simulink model "sampleModel2079"  (R2023a)
settings: Solver=VariableStepAuto  StartTime=0.0  StopTime=10.0  RelTol=1e-3
libraries: hdlsllib x8, simulink x3
settings Model: Creator=user1  LastModifiedBy=user1

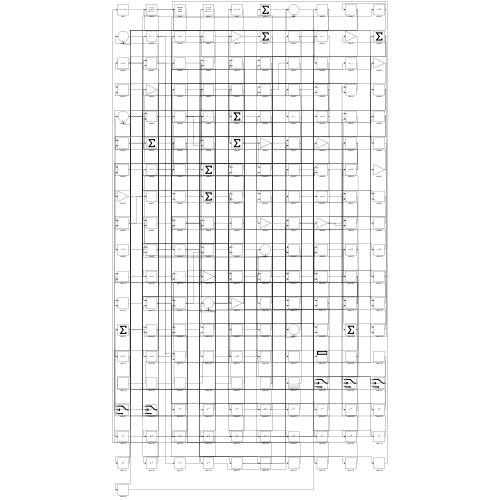
[thumbnail: Simulink's stored preview of the top-level diagram]
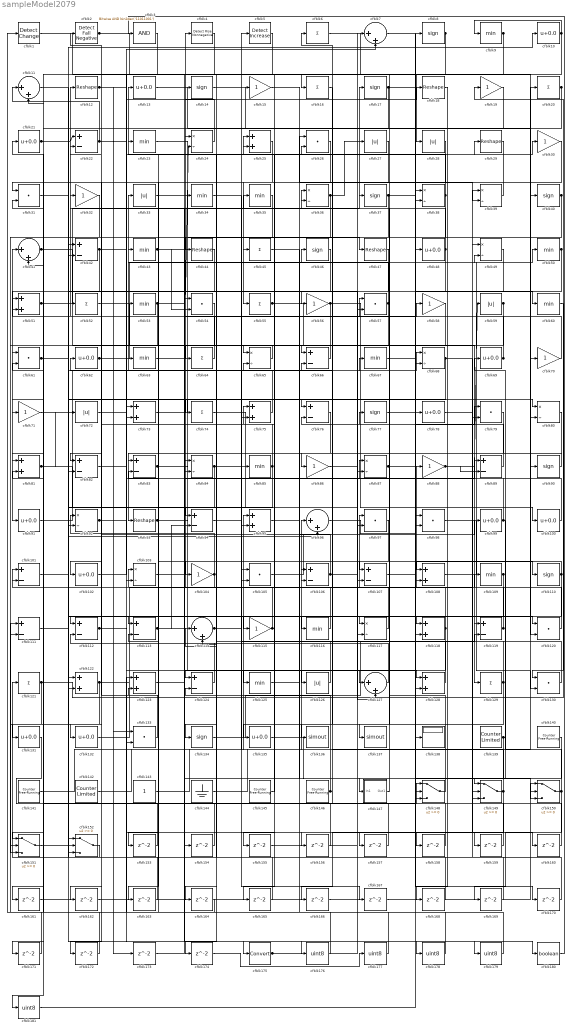
== system sampleModel2079 ==
  cfblk1 : simulink/Logic and Bit Operations/Detect Change  vinit=0  OutDataTypeStr=boolean
      settings: LibrarySourceBlock=|
      | hdlsllib/Logic and Bit
      | Operations/Detect
      | Change
  cfblk{10,13,21,48,62,69,78,91,99..100,102,131..132,135} (14 alike) : Bias  Bias=0.0  SaturateOnIntegerOverflow=off
  cfblk{22,42,66,76,82..83,89,94,101,106..107,111..113,119,124} (16 alike) : Sum  Inputs=+-
  cfblk{24,36,38..39,49,65,68,80,84,87,92,103,117} (13 alike) : Product  Inputs=*/  RndMeth=Zero  SaturateOnIntegerOverflow=on
  cfblk{15,19,30,32,56,58,70..71,86,88,104,115} (12 alike) : Gain
  cfblk{26,31,54,57,61,79,97..98,105,120,130,133} (12 alike) : DotProduct  OutDataTypeStr=Inherit: Inherit via internal rule
  cfblk{25,51,73,75,81,95,108,118,122..123,128} (11 alike) : Sum
  cfblk{9,23,34..35,43,50,53,60,63,67,85,109,116,125} (14 alike) : MinMax
  cfblk{7,11,41,96,114,127} (6 alike) : Sum  Inputs=|++
  cfblk{8,14,17,37,40,46,77,90,110,134} (10 alike) : Signum
  cfblk{12,18,29,44,47,93} (6 alike) : Reshape
  cfblk{6,16,20,45,52,55,64,74,121,129} (10 alike) : Sum  Inputs=+
  cfblk{27..28,33,59,72,126} (6 alike) : Abs  SaturateOnIntegerOverflow=off
  cfblk136 : ToWorkspace  VariableName=simout  SaveFormat=Timeseries  SampleTime=-1
  cfblk137 : ToWorkspace  VariableName=simout  SaveFormat=Timeseries  SampleTime=-1
  cfblk138 : Display
  cfblk139 : hdlsllib/Sources/Counter Limited  uplimit=7  tsamp=-1
  cfblk{140..141,145..146} (4 alike) : hdlsllib/Sources/Counter Free-Running  NumBits=16  tsamp=-1
  cfblk142 : hdlsllib/Sources/Counter Limited  uplimit=7  tsamp=-1
  cfblk143 : Constant  SampleTime=-1
  cfblk144 : Ground
  cfblk147 : Subsystem
      settings: LibrarySourceBlock=|
      | hdlsllib/Ports &
      | Subsystems/Subsystem
  cfblk{148..152} (5 alike) : Switch  SaturateOnIntegerOverflow=off  InputSameDT=off
  cfblk{153..174} (22 alike) : Delay  SampleTime=1
  cfblk175 : DataTypeConversion  SaturateOnIntegerOverflow=off  RndMeth=Floor
  cfblk{176..179,181} (5 alike) : DataTypeConversion  OutDataTypeStr=uint8  SaturateOnIntegerOverflow=off  RndMeth=Floor
  cfblk180 : DataTypeConversion  OutDataTypeStr=boolean  SaturateOnIntegerOverflow=off  RndMeth=Floor
  cfblk2 : hdlsllib/Logic and Bit Operations/Detect Fall Negative  vinit=0  OutDataTypeStr=boolean
  cfblk3 : simulink/Logic and Bit Operations/Bitwise Operator  logicop=AND  UseBitMask=on  BitMask=bin2dec('11011001')  BitMaskRealWorld=Stored Integer
      settings: LibrarySourceBlock=|
      | hdlsllib/Logic and Bit
      | Operations/Bitwise
      | Operator
  cfblk4 : hdlsllib/Logic and Bit Operations/Detect Rise Nonnegative  vinit=0  OutDataTypeStr=boolean
  cfblk5 : simulink/Logic and Bit Operations/Detect Increase  vinit=0.0  OutDataTypeStr=boolean
      settings: LibrarySourceBlock=|
      | hdlsllib/Logic and Bit
      | Operations/Detect
      | Increase
  wires:
  cfblk64/1 -> cfblk12/1
  cfblk76/1 -> cfblk93/1
  cfblk126/1 -> cfblk103/1
  cfblk119/1 -> cfblk97/1, cfblk53/1
  cfblk57/1 -> cfblk33/1, cfblk76/1
  cfblk128/1 -> cfblk62/1
  cfblk70/1 -> cfblk41/1
  cfblk116/1 -> cfblk4/1
  cfblk42/1 -> cfblk91/1, cfblk7/2
  cfblk121/1 -> cfblk19/1, cfblk151/2, cfblk68/2
  cfblk141/1 -> cfblk95/1
  cfblk122/1 -> cfblk88/1, cfblk131/1
  cfblk25/1 -> cfblk112/1
  cfblk48/1 -> cfblk17/1, cfblk135/1
  cfblk23/1 -> cfblk128/1
  cfblk56/1 -> cfblk100/1, cfblk134/1
  cfblk93/1 -> cfblk117/1, cfblk158/1
  cfblk1/1 -> cfblk16/1
  cfblk131/1 -> cfblk148/1
  cfblk40/1 -> cfblk137/1, cfblk151/3
  cfblk89/1 -> cfblk6/1
  cfblk102/1 -> cfblk87/1
  cfblk108/1 -> cfblk50/1
  cfblk88/1 -> cfblk59/1, cfblk89/2
  cfblk65/1 -> cfblk64/1
  cfblk74/1 -> cfblk117/2
  cfblk10/1 -> cfblk9/1, cfblk11/2
  cfblk105/1 -> cfblk98/1
  cfblk38/1 -> cfblk13/1, cfblk44/1, cfblk151/1
  cfblk110/1 -> cfblk115/1, cfblk104/1
  cfblk30/1 -> cfblk55/1
  cfblk73/1 -> cfblk80/1
  cfblk115/1 -> cfblk24/1, cfblk65/2
  cfblk17/1 -> cfblk81/1, cfblk150/2
  cfblk147/1(Out1) -> cfblk77/1
  cfblk117/1 -> cfblk81/2
  cfblk79/1 -> cfblk86/1
  cfblk148/1 -> cfblk32/1
  cfblk118/1 -> cfblk46/1, cfblk174/1
  cfblk53/1 -> cfblk24/2, cfblk161/1
  cfblk130/1 -> cfblk25/1
  cfblk12/1 -> cfblk73/1, cfblk173/1
  cfblk80/1 -> cfblk108/1
  cfblk149/1 -> cfblk106/1, cfblk166/1
  cfblk69/1 -> cfblk57/1, cfblk26/2
  cfblk41/1 -> cfblk129/1, cfblk56/1, cfblk116/1
  cfblk72/1 -> cfblk67/1
  cfblk27/1 -> cfblk102/1
  cfblk135/1 -> cfblk147/1(In1)
  cfblk112/1 -> cfblk156/1, cfblk157/1
  cfblk51/1 -> cfblk5/1, cfblk179/1
  cfblk6/1 -> cfblk28/1
  cfblk14/1 -> cfblk78/1
  cfblk127/1 -> cfblk112/2
  cfblk99/1 -> cfblk35/1, cfblk149/1
  cfblk26/1 -> cfblk73/2
  cfblk129/1 -> cfblk76/2, cfblk155/1
  cfblk66/1 -> cfblk61/1
  cfblk90/1 -> cfblk83/1
  cfblk124/1 -> cfblk83/2
  cfblk54/1 -> cfblk111/2
  cfblk36/1 -> cfblk132/1, cfblk27/1
  cfblk120/1 -> cfblk101/1
  cfblk33/1 -> cfblk47/1
  cfblk101/1 -> cfblk10/1
  cfblk143/1 -> cfblk96/1
  cfblk96/1 -> cfblk98/2
  cfblk91/1 -> cfblk43/1
  cfblk20/1 -> cfblk126/1, cfblk120/2
  cfblk123/1 -> cfblk175/1
  cfblk21/1 -> cfblk22/1, cfblk96/2
  cfblk139/1 -> cfblk69/1, cfblk149/2
  cfblk144/1 -> cfblk40/1
  cfblk16/1 -> cfblk66/1
  cfblk106/1 -> cfblk2/1, cfblk89/1
  cfblk32/1 -> cfblk152/2
  cfblk114/1 -> cfblk15/1, cfblk37/1, cfblk119/2
  cfblk68/1 -> cfblk80/2, cfblk82/2
  cfblk107/1 -> cfblk38/2
  cfblk132/1 -> cfblk49/1
  cfblk60/1 -> cfblk130/1
  cfblk146/1 -> cfblk84/1, cfblk106/2
  cfblk19/1 -> cfblk125/1
  cfblk7/1 -> cfblk60/1
  cfblk95/1 -> cfblk118/1
  cfblk13/1 -> cfblk70/1
  cfblk100/1 -> cfblk34/1
  cfblk55/1 -> cfblk148/2, cfblk150/3
  cfblk22/1 -> cfblk11/1, cfblk128/2, cfblk133/1
  cfblk43/1 -> cfblk138/1, cfblk97/2, cfblk54/2, cfblk149/3
  cfblk67/1 -> cfblk108/2
  cfblk46/1 -> cfblk51/1
  cfblk85/1 -> cfblk22/2, cfblk152/3
  cfblk5/1 -> cfblk71/1
  cfblk29/1 -> cfblk136/1
  cfblk62/1 -> cfblk20/1, cfblk176/1
  cfblk111/1 -> cfblk113/1
  cfblk75/1 -> cfblk23/1
  cfblk133/1 -> cfblk92/1
  cfblk145/1 -> cfblk75/1
  cfblk49/1 -> cfblk103/2
  cfblk98/1 -> cfblk130/2
  cfblk31/1 -> cfblk95/2
  cfblk15/1 -> cfblk39/2
  cfblk104/1 -> cfblk52/1, cfblk101/2
  cfblk35/1 -> cfblk124/1
  cfblk142/1 -> cfblk85/1
  cfblk2/1 -> cfblk90/1, cfblk84/2
  cfblk151/1 -> cfblk68/1
  cfblk152/1 -> cfblk121/1
  cfblk134/1 -> cfblk48/1
  cfblk86/1 -> cfblk120/1
  cfblk52/1 -> cfblk65/1
  cfblk50/1 -> cfblk127/1, cfblk82/1
  cfblk87/1 -> cfblk79/1, cfblk110/1
  cfblk24/1 -> cfblk14/1
  cfblk113/1 -> cfblk36/1, cfblk94/2
  cfblk81/1 -> cfblk105/1, cfblk72/1
  cfblk59/1 -> cfblk105/2, cfblk162/1
  cfblk11/1 -> cfblk74/1
  cfblk47/1 -> cfblk114/2
  cfblk140/1 -> cfblk148/3
  cfblk84/1 -> cfblk92/2, cfblk167/1
  cfblk83/1 -> cfblk58/1, cfblk127/2, cfblk180/1
  cfblk37/1 -> cfblk30/1, cfblk45/1
  cfblk39/1 -> cfblk31/1
  cfblk109/1 -> cfblk119/1, cfblk122/2
  cfblk9/1 -> cfblk107/1, cfblk133/2
  cfblk125/1 -> cfblk99/1
  cfblk45/1 -> cfblk79/2
  cfblk94/1 -> cfblk49/2
  cfblk150/1 -> cfblk109/1, cfblk169/1
  cfblk8/1 -> cfblk94/1, cfblk165/1
  cfblk71/1 -> cfblk42/2
  cfblk61/1 -> cfblk75/2, cfblk21/1
  cfblk82/1 -> cfblk25/2
  cfblk92/1 -> cfblk18/1, cfblk29/1
  cfblk97/1 -> cfblk153/1
  cfblk153/1 -> cfblk61/2
  cfblk103/1 -> cfblk154/1
  cfblk154/1 -> cfblk42/1
  cfblk155/1 -> cfblk87/2
  cfblk156/1 -> cfblk41/2
  cfblk157/1 -> cfblk66/2
  cfblk158/1 -> cfblk36/2
  cfblk34/1 -> cfblk159/1
  cfblk159/1 -> cfblk113/2
  cfblk78/1 -> cfblk160/1
  cfblk160/1 -> cfblk114/1
  cfblk161/1 -> cfblk107/2
  cfblk162/1 -> cfblk118/2
  cfblk28/1 -> cfblk163/1
  cfblk163/1 -> cfblk122/1
  cfblk58/1 -> cfblk164/1
  cfblk164/1 -> cfblk1/1
  cfblk165/1 -> cfblk124/2
  cfblk166/1 -> cfblk38/1
  cfblk167/1 -> cfblk150/1
  cfblk18/1 -> cfblk168/1
  cfblk168/1 -> cfblk152/1
  cfblk169/1 -> cfblk31/2
  cfblk77/1 -> cfblk170/1
  cfblk170/1 -> cfblk39/1
  cfblk4/1 -> cfblk171/1
  cfblk171/1 -> cfblk111/1
  cfblk44/1 -> cfblk172/1
  cfblk172/1 -> cfblk51/2
  cfblk173/1 -> cfblk54/1
  cfblk175/1 -> cfblk7/1, cfblk57/2
  cfblk176/1 -> cfblk123/1
  cfblk174/1 -> cfblk177/1
  cfblk177/1 -> cfblk123/2
  cfblk63/1 -> cfblk178/1
  cfblk178/1 -> cfblk26/1
  cfblk179/1 -> cfblk63/1
  cfblk180/1 -> cfblk3/1
  cfblk3/1 -> cfblk181/1
  cfblk181/1 -> cfblk8/1

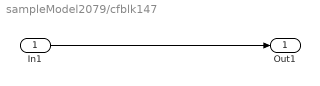
== system sampleModel2079/cfblk147 ==
  In1 : Inport
  Out1 : Outport
  wires:
  In1/1 -> Out1/1
